simulink model "Atomic_Subsystem"  (R2020b)
settings: Solver=FixedStepAuto  StartTime=0.0  StopTime=10.0  FixedStep=0.2  RelTol=1e-3
settings Model: Creator=Admin  LastModifiedBy=Admin
settings DataIOCC: SaveOutput=off  SaveTime=off

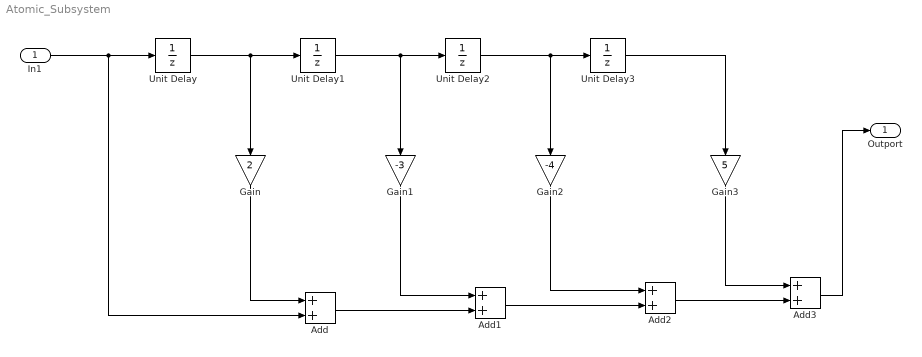
== system Atomic_Subsystem ==
  In1 : Inport  OutDataTypeStr=double  PortDimensions=1
  Add{,1..3} (4 alike) : Sum
  Gain : Gain  Gain=2
  Gain1 : Gain  Gain=-3
  Gain2 : Gain  Gain=-4
  Gain3 : Gain  Gain=5
  Unit Delay{,1..3} (4 alike) : UnitDelay  SampleTime=-1  HasFrameUpgradeWarning=on
  Outport : Outport  OutDataTypeStr=double  PortDimensions=1  SampleTime=[0.20000000000000001,0]
  wires:
  Add2/1 -> Add3/2
  Add/1 -> Add1/2
  Add1/1 -> Add2/2
  Gain1/1 -> Add1/1
  Gain/1 -> Add/1
  Gain2/1 -> Add2/1
  Unit Delay1/1 -> Unit Delay2/1, Gain1/1
  Unit Delay/1 -> Unit Delay1/1, Gain/1
  Unit Delay3/1 -> Gain3/1
  Unit Delay2/1 -> Unit Delay3/1, Gain2/1
  Gain3/1 -> Add3/1
  In1/1 -> Unit Delay/1, Add/2
  Add3/1 -> Outport/1
